simulink model "EX_Gain_1mdl"  (Simulink 4.00)
settings: Solver=ode45  StartTime=0.0  StopTime=10.0  RelTol=1e-3
settings Model: LastModifiedBy=Администратор

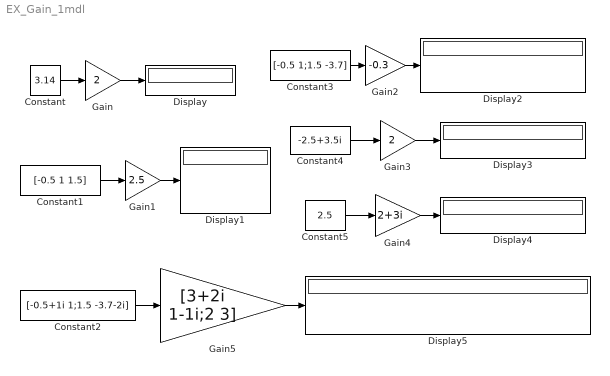
== system EX_Gain_1mdl ==
  Constant : Constant  Value=3.14
  Constant1 : Constant  Value=[-0.5 1 1.5]
  Constant2 : Constant  Value=[-0.5+1i 1;1.5 -3.7-2i]  VectorParams1D=off
  Constant3 : Constant  Value=[-0.5 1;1.5 -3.7]  VectorParams1D=off
  Constant4 : Constant  Value=-2.5+3.5i
  Constant5 : Constant  Value=2.5
  Display{,1..5} (6 alike) : Display
      settings: Format=short
  Gain : Gain  Gain=2  Multiplication=Element-wise(K.*u)  SaturateOnIntegerOverflow=on
  Gain1 : Gain  Gain=2.5  Multiplication=Element-wise(K.*u)  SaturateOnIntegerOverflow=on
  Gain2 : Gain  Gain=-0.3  Multiplication=Element-wise(K.*u)  SaturateOnIntegerOverflow=on
  Gain3 : Gain  Gain=2  Multiplication=Element-wise(K.*u)  SaturateOnIntegerOverflow=on
  Gain4 : Gain  Gain=2+3i  Multiplication=Element-wise(K.*u)  SaturateOnIntegerOverflow=on
  Gain5 : Gain  Gain=[3+2i 1-1i;2 3]  Multiplication=Element-wise(K.*u)  SaturateOnIntegerOverflow=on
  wires:
  Constant/1 -> Gain/1
  Gain/1 -> Display/1
  Gain1/1 -> Display1/1
  Constant1/1 -> Gain1/1
  Constant3/1 -> Gain2/1
  Gain2/1 -> Display2/1
  Constant4/1 -> Gain3/1
  Gain3/1 -> Display3/1
  Constant5/1 -> Gain4/1
  Gain4/1 -> Display4/1
  Constant2/1 -> Gain5/1
  Gain5/1 -> Display5/1
